simulink model "week2problem3"  (R2020b)
settings: Solver=VariableStepAuto  StartTime=0.0  StopTime=10.0  RelTol=1e-3
values from neighbouring files (symbols this model uses):
  b = 50    [thirdprblm.m]
  m = 1000    [thirdprblm.m]
settings Model: Creator=Admin  LastModifiedBy=Admin

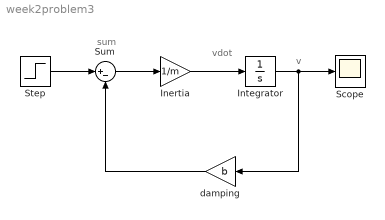
== system week2problem3 ==
  note: sum
  note: v
  note: vdot
  Inertia : Gain  Gain=1/m
  Integrator : Integrator
  Scope : Scope
  Step : Step  After=u  SampleTime=0
  Sum : Sum  Inputs=|+-
  damping : Gain  Gain=b
  wires:
  Sum/1 -> Inertia/1
  Inertia/1 -> Integrator/1
  Integrator/1 -> damping/1, Scope/1
  damping/1 -> Sum/2
  Step/1 -> Sum/1
